simulink model "sampleModel21"  (R2021b)
settings: Solver=VariableStepAuto  StartTime=0.0  StopTime=10.0  RelTol=1e-3
undefined symbols (not defined in the file or in its folder): DiscIntNeverNeededParam, Newton, Raphson
libraries: simulink x6
settings Model: Creator=user  LastModifiedBy=user

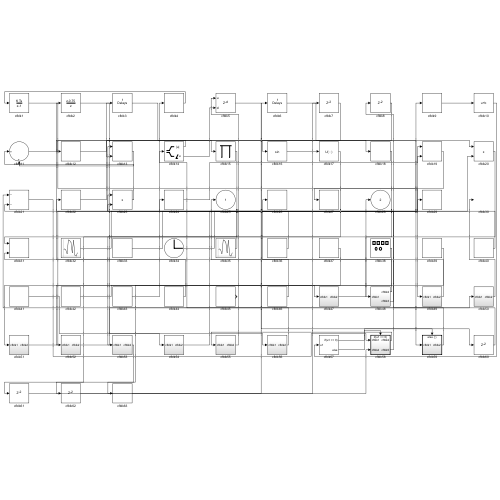
[thumbnail: Simulink's stored preview of the top-level diagram]
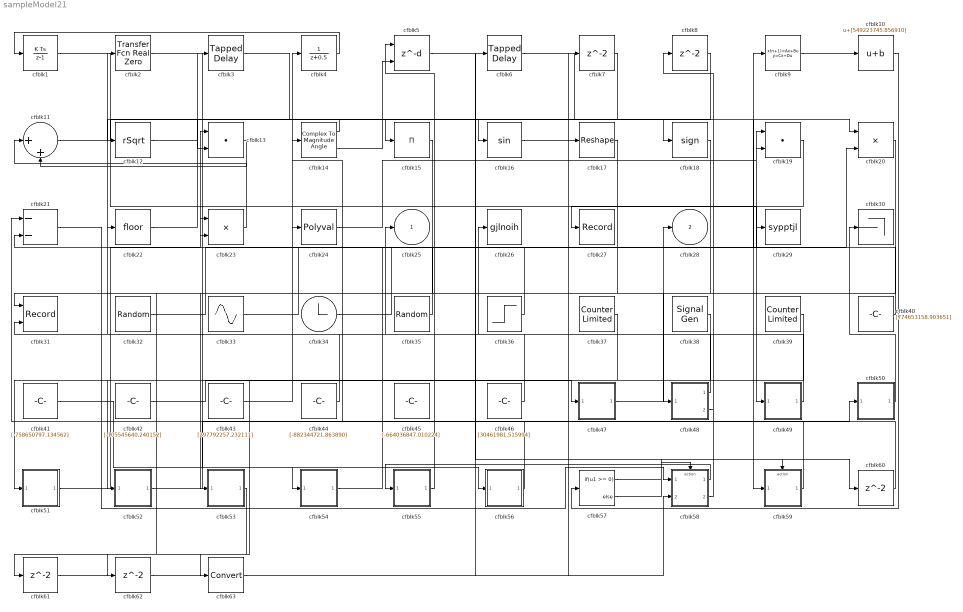
== system sampleModel21 ==
  cfblk1 : DiscreteIntegrator  ICPrevOutput=DiscIntNeverNeededParam  ICPrevScaledInput=DiscIntNeverNeededParam
  cfblk10 : Bias  Bias=[549223745.856910]
  cfblk11 : Sum  Inputs=|++
  cfblk12 : Sqrt  Operator=rSqrt  AlgorithmType=Newton-Raphson  SaturateOnIntegerOverflow=on
  cfblk13 : DotProduct  InputSameDT=on  OutDataTypeStr=Inherit: Inherit via internal rule
  cfblk14 : ComplexToMagnitudeAngle
  cfblk15 : Product  Inputs=*
  cfblk16 : Trigonometry
  cfblk17 : Reshape
  cfblk18 : Signum
  cfblk19 : DotProduct  InputSameDT=on  OutDataTypeStr=Inherit: Inherit via internal rule
  cfblk2 : simulink/Discrete/Transfer Fcn Real Zero  ZeroZ=0.75  ICPrevInput=0.0  DoSatur=off
      settings: SourceProductBaseCode=SL
  cfblk20 : Product  Inputs=**
  cfblk21 : Sum  Inputs=--
  cfblk22 : Rounding
  cfblk23 : Product
  cfblk24 : Polyval  Coefs=[ +2.081618890e-019, -1.441693666e-014, +4.719686976e-010, -8.536869453e-006, +1.621573104e-001, -8.087801117e+001 ]
  cfblk26 : ToWorkspace  VariableName=gjlnoih  SaveFormat=Timeseries  SampleTime=-1
  cfblk27 : Record  FileSettingsInternal="{\"entries\":[{\"content\":{\"excelSettings\":{\"content\":{},\"type\":\"Streamout.ExcelSettings\"}},\"type\":\"Streamout.FileSettingStorage\",\"uuid\":\"06ae0355-d5c6-42cb-9c90-f28d0b9c9483\"}],\"packageUris\":[\"http://schema.mathworks.com/mf0/streamout_blocks/R2020a\"],\"version\":\"1.0\"}"  SignalsInternal="{\"entries\":[{\"content\":{\"signals\":[{\"content\":{\"blockPath\":[\"sampleModel21/cfblk27\"],\"channel\":[],\"dimensions\":[1],\"domain\":\"sampleModel21/cfblk27\",\"lineColor\":\"#7e2f8e\",\"plots\":[1],\"port\":1,\"sid\":[\"\"],\"signalID\":857,\"signalName\":\"cfblk19\"},\"type\":\"RecordBlkView.Signal\",\"uuid\":\"550456b8-a3c5-4e99-9496-18ba5b3ce816\"}]},\"type\":\"RecordBlkView.InputSignals\",\"uuid\":\"227f541e-70fe-4312-9297-2dd5238bfc09\"}],\"packageUris\":[\"http://schema.mathworks.com/mf0/streamout_blocks/R2020a\"],\"version\":\"1.0\"}"  VisualizationBindings="{\"sparklinesplugin\":{\"info\":[{\"bindingParametersList\":[],\"subplotID\":1}]}}"
  cfblk29 : ToWorkspace  VariableName=sypptjl  SaveFormat=Timeseries  SampleTime=-1
  cfblk3 : simulink/Discrete/Tapped Delay  vinit=0.0  samptime=-1  NumDelays=1  DelayOrder=Oldest  includeCurrent=off
  cfblk30 : Terminator
  cfblk31 : Record  FileSettingsInternal="{\"entries\":[{\"content\":{\"excelSettings\":{\"content\":{},\"type\":\"Streamout.ExcelSettings\"}},\"type\":\"Streamout.FileSettingStorage\",\"uuid\":\"4404ca33-d5d5-4be6-a275-f212b1ac5b68\"}],\"packageUris\":[\"http://schema.mathworks.com/mf0/streamout_blocks/R2020a\"],\"version\":\"1.0\"}"  Layout=[1 1]  SignalsInternal="{\"entries\":[{\"content\":{\"signals\":[{\"content\":{\"blockPath\":[\"sampleModel21/cfblk31\"],\"channel\":[],\"dimensions\":[1],\"domain\":\"sampleModel21/cfblk31\",\"lineColor\":\"#a2142f\",\"plots\":[1],\"port\":1,\"sid\":[\"\"],\"signalID\":861,\"signalName\":\"cfblk20\"},\"type\":\"RecordBlkView.Signal\",\"uuid\":\"5181162e-a2c5-45a1-a0af-fcb2aa090d6f\"},{\"content\":{\"blockPath\":[\"sampleModel21/cfblk31\"],\"channel\":[],\"dimensions\":[1],\"domain\":\"sampleModel21/cfblk31\",\"lineColor\":\"#139fff\",\"plots\":[1],\"port\":2,\"sid\":[\"\"],\"signalID\":865,\"signalName\":\"cfblk46\"},\"type\":\"RecordBlkView.Signal\",\"uuid\":\"9564f83f-bdb7-4cc9-95b8-b8a620c636c1\"}]},\"type\":\"RecordBlkView.InputSignals\",\"uuid\":\"d3e53b74-13ce-485c-bd9d-9082c0f77247\"}],\"packageUris\":[\"http://schema.mathworks.com/mf0/streamout_blocks/R2020a\"],\"version\":\"1.0\"}"  VisualizationBindings="{\"xyplotplugin\":{\"info\":[{\"series\":[{\"bindingParametersList\":[{\"parameter\":\"X-Axis\",\"signalID\":861,\"signalName\":\"cfblk20\"},{\"parameter\":\"Y-Axis\",\"signalID\":865,\"signalName\":\"cfblk46\"}],\"seriesID\":12145}],\"subplotID\":1}]}}"  CompatibilityTag=XY
  cfblk32 : RandomNumber  Mean=[1875.112904]  Variance=[92871.083530]  Seed=[450787807.000000]  SampleTime=0.1
  cfblk33 : Sin  Amplitude=[274869736.107470]  Bias=[-81272284.351688]  SampleTime=0
  cfblk34 : Clock
  cfblk35 : RandomNumber  Mean=[10754.891883]  Variance=[4123.265892]  Seed=[802202179.000000]  SampleTime=0.1
  cfblk36 : Step  Time=[33.000000]  Before=[-599344810.418858]  After=[-970827253.016853]  SampleTime=0
  cfblk37 : simulink/Sources/Counter Limited  uplimit=[763.000000]  tsamp=-1
  cfblk38 : SignalGenerator  WaveForm=square  Amplitude=[135023519.724701]
  cfblk39 : simulink/Sources/Counter Limited  uplimit=[734.000000]  tsamp=-1
  cfblk4 : DiscreteTransferFcn  SampleTime=1
  cfblk40 : Constant  Value=[774653158.903651]  SampleTime=1
  cfblk41 : Constant  Value=[-758650797.134562]  SampleTime=1
  cfblk42 : Constant  Value=[-105545640.240152]  SampleTime=1
  cfblk43 : Constant  Value=[297792257.232111]  SampleTime=1
  cfblk44 : Constant  Value=[-882344721.863890]  SampleTime=1
  cfblk45 : Constant  Value=[-664036847.010224]  SampleTime=1
  cfblk46 : Constant  Value=[30461981.515994]  SampleTime=1
  cfblk47 : Subsystem
  cfblk48 : Subsystem
  cfblk49 : Subsystem
  cfblk5 : Delay  DelayLengthSource=Input port  SampleTime=1
      settings: InputPortMap=u0,p1
  cfblk50 : Subsystem
  cfblk51 : Subsystem
  cfblk52 : Subsystem
  cfblk53 : Subsystem
  cfblk54 : Subsystem
  cfblk55 : Subsystem
  cfblk56 : Subsystem
  cfblk57 : If  IfExpression=u1 >= 0  SampleTime=1
  cfblk58 : Subsystem  TreatAsAtomicUnit=on
  cfblk59 : Subsystem  TreatAsAtomicUnit=on
  cfblk6 : simulink/Discrete/Tapped Delay  vinit=0.0  samptime=-1  NumDelays=1  DelayOrder=Oldest  includeCurrent=off
  cfblk{7..8,60..62} (5 alike) : Delay  SampleTime=1
  cfblk63 : DataTypeConversion
  cfblk9 : DiscreteStateSpace
  cfblk25 : Outport
  cfblk28 : Outport  Port=2
  wires:
  cfblk58/1(cfblk2) -> cfblk55/1(cfblk1)
  cfblk16/1 -> cfblk17/1
  cfblk48/1(cfblk2) -> cfblk25/1
  cfblk52/1(cfblk2) -> cfblk50/1(cfblk1)
  cfblk1/1 -> cfblk49/1(cfblk1)
  cfblk2/1 -> cfblk56/1(cfblk1)
  cfblk44/1 -> cfblk2/1
  cfblk35/1 -> cfblk22/1
  cfblk9/1 -> cfblk10/1
  cfblk6/1 -> cfblk59/1(cfblk1)
  cfblk43/1 -> cfblk4/1
  cfblk11/1 -> cfblk15/1
  cfblk47/1(cfblk2) -> cfblk28/1
  cfblk18/1 -> cfblk48/1(cfblk1)
  cfblk24/1 -> cfblk19/1
  cfblk49/1(cfblk2) -> cfblk26/1
  cfblk10/1 -> cfblk57/1
  cfblk23/1 -> cfblk11/1
  cfblk21/1 -> cfblk58/1(cfblk1)
  cfblk15/1 -> cfblk53/1(cfblk1)
  cfblk59/1(cfblk2) -> cfblk8/1
  cfblk41/1 -> cfblk54/1(cfblk1)
  cfblk32/1 -> cfblk19/2
  cfblk50/1(cfblk2) -> cfblk30/1
  cfblk4/1 -> cfblk1/1
  cfblk51/1(cfblk2) -> cfblk13/1
  cfblk58/2(cfblk5) -> cfblk23/1
  cfblk7/1 -> cfblk13/2
  cfblk38/1 -> cfblk51/1(cfblk1)
  cfblk14/1 -> cfblk12/1
  cfblk8/1 -> cfblk16/1
  cfblk19/1 -> cfblk27/1
  cfblk20/1 -> cfblk31/1
  cfblk12/1 -> cfblk18/1
  cfblk22/1 -> cfblk3/1
  cfblk13/1 -> cfblk11/2
  cfblk3/1 -> cfblk20/1
  cfblk37/1 -> cfblk52/1(cfblk1)
  cfblk40/1 -> cfblk24/1
  cfblk46/1 -> cfblk31/2
  cfblk36/1 -> cfblk23/2
  cfblk33/1 -> cfblk9/1
  cfblk56/1(cfblk2) -> cfblk14/1
  cfblk55/1(cfblk2) -> cfblk5/1
  cfblk48/2(cfblk3) -> cfblk21/2
  cfblk34/1 -> cfblk20/2
  cfblk42/1 -> cfblk47/1(cfblk1)
  cfblk54/1(cfblk2) -> cfblk29/1
  cfblk14/2 -> cfblk5/2
  cfblk57/1 -> cfblk58/Action
  cfblk57/2 -> cfblk59/Action
  cfblk5/1 -> cfblk60/1
  cfblk60/1 -> cfblk21/1
  cfblk53/1(cfblk2) -> cfblk61/1
  cfblk61/1 -> cfblk58/2(cfblk4)
  cfblk17/1 -> cfblk62/1
  cfblk62/1 -> cfblk6/1
  cfblk39/1 -> cfblk63/1
  cfblk63/1 -> cfblk7/1

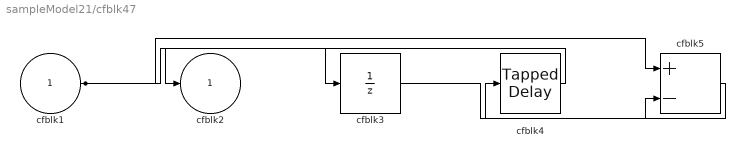
== system sampleModel21/cfblk47 ==
  cfblk1 : Inport
  cfblk3 : UnitDelay  HasFrameUpgradeWarning=on
  cfblk4 : simulink/Discrete/Tapped Delay  vinit=0.0  samptime=-1  NumDelays=1  DelayOrder=Oldest  includeCurrent=off
  cfblk5 : Sum  Inputs=+-
  cfblk2 : Outport
  wires:
  cfblk4/1 -> cfblk2/1
  cfblk1/1 -> cfblk5/1, cfblk3/1
  cfblk5/1 -> cfblk4/1
  cfblk3/1 -> cfblk5/2

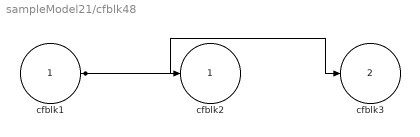
== system sampleModel21/cfblk48 ==
  cfblk1 : Inport
  cfblk2 : Outport
  cfblk3 : Outport  Port=2
  wires:
  cfblk1/1 -> cfblk3/1, cfblk2/1

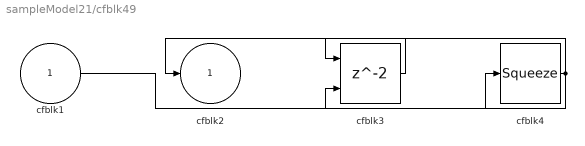
== system sampleModel21/cfblk49 ==
  cfblk1 : Inport
  cfblk3 : Delay  ShowEnablePort=on  SampleTime=1
      settings: InputPortMap=u0,e6
  cfblk4 : Squeeze
  cfblk2 : Outport
  wires:
  cfblk3/1 -> cfblk2/1
  cfblk1/1 -> cfblk4/1
  cfblk4/1 -> cfblk3/1, cfblk3/2

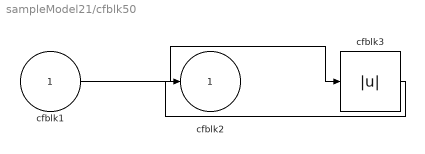
== system sampleModel21/cfblk50 ==
  cfblk1 : Inport
  cfblk3 : Abs
  cfblk2 : Outport
  wires:
  cfblk1/1 -> cfblk3/1
  cfblk3/1 -> cfblk2/1

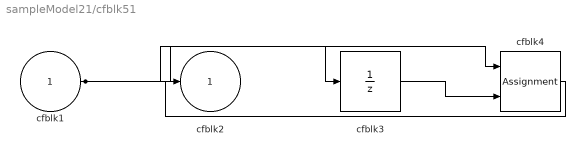
== system sampleModel21/cfblk51 ==
  cfblk1 : Inport
  cfblk3 : UnitDelay  HasFrameUpgradeWarning=on
  cfblk4 : Assignment  DiagnosticForDimensions=Warning  IndexOptions=Index vector (dialog)  Indices=1  OutputSizes=1
  cfblk2 : Outport
  wires:
  cfblk1/1 -> cfblk4/1, cfblk3/1
  cfblk3/1 -> cfblk4/2
  cfblk4/1 -> cfblk2/1

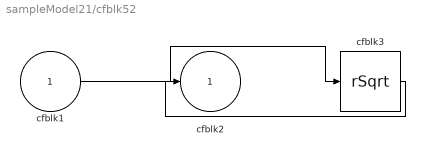
== system sampleModel21/cfblk52 ==
  cfblk1 : Inport
  cfblk3 : Sqrt  Operator=rSqrt  AlgorithmType=Newton-Raphson  SaturateOnIntegerOverflow=on
  cfblk2 : Outport
  wires:
  cfblk1/1 -> cfblk3/1
  cfblk3/1 -> cfblk2/1

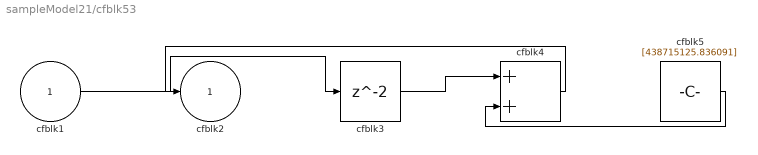
== system sampleModel21/cfblk53 ==
  cfblk1 : Inport
  cfblk3 : Delay  SampleTime=1
  cfblk4 : Sum
  cfblk5 : Constant  Value=[438715125.836091]  SampleTime=1
  cfblk2 : Outport
  wires:
  cfblk3/1 -> cfblk4/1
  cfblk5/1 -> cfblk4/2
  cfblk1/1 -> cfblk3/1
  cfblk4/1 -> cfblk2/1

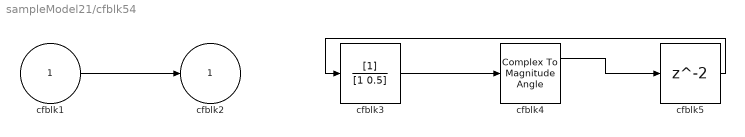
== system sampleModel21/cfblk54 ==
  cfblk1 : Inport
  cfblk3 : DiscreteFilter  SampleTime=1
  cfblk4 : ComplexToMagnitudeAngle
  cfblk5 : Delay  SampleTime=1
  cfblk2 : Outport
  wires:
  cfblk1/1 -> cfblk2/1
  cfblk3/1 -> cfblk4/1
  cfblk4/1 -> cfblk5/1
  cfblk5/1 -> cfblk3/1

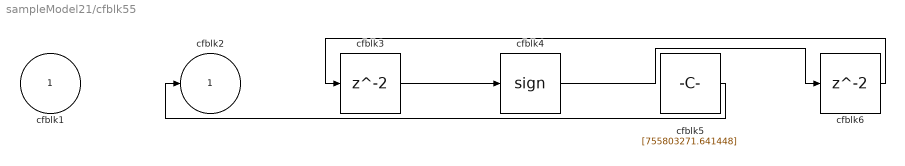
== system sampleModel21/cfblk55 ==
  cfblk1 : Inport
  cfblk3 : Delay  SampleTime=1
  cfblk4 : Signum
  cfblk5 : Constant  Value=[755803271.641448]  SampleTime=1
  cfblk6 : Delay  SampleTime=1
  cfblk2 : Outport
  wires:
  cfblk5/1 -> cfblk2/1
  cfblk3/1 -> cfblk4/1
  cfblk4/1 -> cfblk6/1
  cfblk6/1 -> cfblk3/1

== system sampleModel21/cfblk56 ==
  cfblk1 : Inport
  cfblk3 : Math  Operator=log10  SaturateOnIntegerOverflow=on
  cfblk2 : Outport
  wires:
  cfblk1/1 -> cfblk3/1
  cfblk3/1 -> cfblk2/1

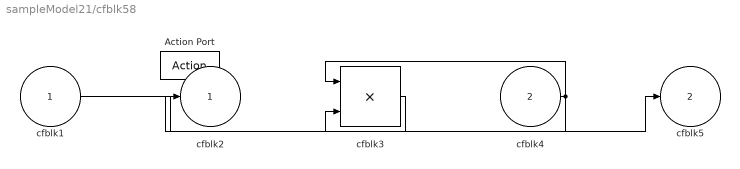
== system sampleModel21/cfblk58 ==
  cfblk1 : Inport
  cfblk4 : Inport  Port=2
  Action Port : ActionPort  ActionPortLabel=if(u1 >= 0)
  cfblk3 : Product  Inputs=**
  cfblk2 : Outport
  cfblk5 : Outport  Port=2
  wires:
  cfblk1/1 -> cfblk5/1
  cfblk4/1 -> cfblk3/1, cfblk3/2
  cfblk3/1 -> cfblk2/1

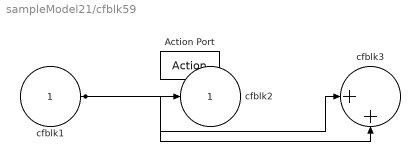
== system sampleModel21/cfblk59 ==
  cfblk1 : Inport
  Action Port : ActionPort  ActionPortLabel=else
  cfblk3 : Sum  Inputs=|++
  cfblk2 : Outport
  wires:
  cfblk1/1 -> cfblk2/1, cfblk3/1, cfblk3/2
